simulink model "penduleBF"  (R2012b)
settings: Solver=ode45  StartTime=0.0  StopTime=15  MaxStep=0.01  RelTol=1e-3  AbsTol=1e-3
values from neighbouring files (symbols this model uses):
  Adc = Ad-(Bd*Kcd)-(Kod*Cd)    [Synthese_Obs_Contr_Pendule.m]
  Bdc = Kod    [Synthese_Obs_Contr_Pendule.m]
  Cdc = Kcd    [Synthese_Obs_Contr_Pendule.m]
  Ddc = [0,0]    [Synthese_Obs_Contr_Pendule.m]
  Tech = 0.01    [Synthese_Obs_Contr_Pendule.m]
settings Model: ExtModeTrigMode=oneshot  ExtModeArmWhenConnect=off  Creator=ArbenCela  LastModifiedBy=lalinden
settings DataIOCC: LimitDataPoints=off  SignalLoggingSaveFormat=ModelDataLogs  SaveOutput=off  SaveTime=off
settings OptimizationCC: BooleanDataType=off  ExpressionDepthLimit=128  InitFltsAndDblsToZero=on
settings DebuggingCC: SaveWithParameterizedLinksMsg=none  SignalResolutionControl=TryResolveAllWithWarning  SolverPrmCheckMsg=none  MultiTaskDSMMsg=warning  MultiTaskCondExecSysMsg=none  FcnCallInpInsideContextMsg=UseLocalSettings  StateNameClashWarn=none  StrictBusMsg=None
settings HardwareCC: TargetUnknown=on
settings RTWCC: IncludeERTFirstTime=on
settings CodeAppCC: CustomSymbolStrType=$N$R$M_T  InternalIdentifier=Shortened
settings GRTTargetCC: TargetFcnLib=ansi_tfl_tmw.mat  CodeReplacementLibrary=None  CombineOutputUpdateFcns=off  CPPClassGenCompliant=on  GRTInterface=on

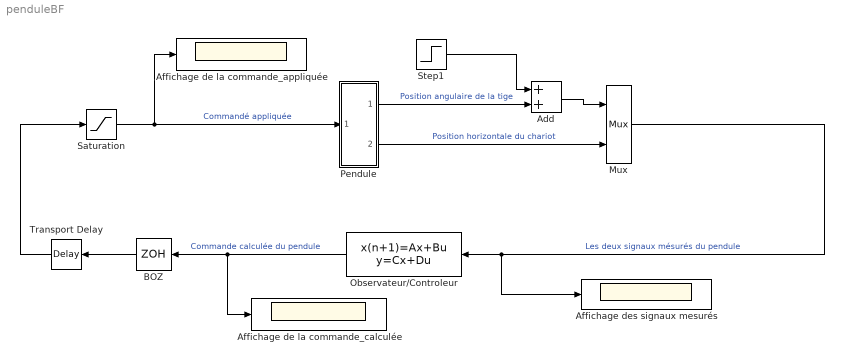
== system penduleBF ==
  Add : Sum
  Affichage de la commande_appliquée : Scope
      settings: YMin=2e+008  YMax=5.75e+008  SaveName=ScopeData2
  Affichage de la commande_calculée : Scope
      settings: YMin=2e+008  YMax=5.75e+008
  Affichage des signaux mesurés : Scope
      settings: YMin=-250000  YMax=1.75e+006
  BOZ : ZeroOrderHold  SampleTime=Tech
  Mux : Mux  Inputs=2
  Observateur/Controleur : DiscreteStateSpace  A=Adc  B=Bdc  C=-Cdc  D=Ddc  X0=[0;0;0;0]  SampleTime=Tech
  Pendule : Subsystem
  Saturation : Saturate  UpperLimit=10  LowerLimit=-10
  Step1 : Step  Time=2  After=0.02  SampleTime=0
  Transport Delay : TransportDelay  DelayTime=0.005
  wires:
  Pendule/2(out_2) -> Mux/2  "Position horizontale du chariot"
  Observateur/Controleur/1 -> Affichage de la commande_calculée/1, BOZ/1  "Commande calculée du pendule"
  Mux/1 -> Observateur/Controleur/1, Affichage des signaux mesurés/1  "Les deux signaux mésurés du pendule"
  Saturation/1 -> Pendule/1(in_1), Affichage de la commande_appliquée/1  "Commandé appliquée"
  Pendule/1(out_1) -> Add/2  "Position angulaire de la tige"
  Add/1 -> Mux/1
  BOZ/1 -> Transport Delay/1
  Transport Delay/1 -> Saturation/1
  Step1/1 -> Add/1

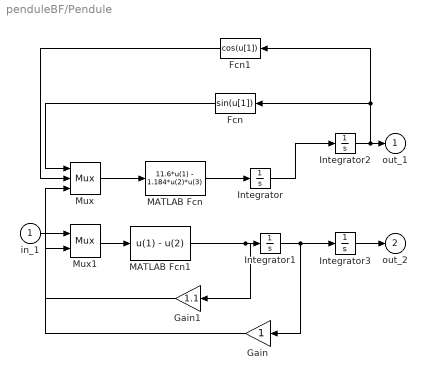
== system penduleBF/Pendule ==
  in_1 : Inport
  Fcn : Fcn
  Fcn1 : Fcn  Expr=cos(u[1])
  Gain : Gain  SaturateOnIntegerOverflow=on  OutDataTypeStr=Inherit: Same as input  ParamDataTypeStr=Inherit: Same as input
  Gain1 : Gain  Gain=1.1  SaturateOnIntegerOverflow=on  OutDataTypeStr=Inherit: Same as input  ParamDataTypeStr=Inherit: Same as input
  Integrator : Integrator
  Integrator1 : Integrator
  Integrator2 : Integrator  InitialCondition=0.1
  Integrator3 : Integrator
  MATLAB Fcn : MATLABFcn  MATLABFcn=11.6*u(1) - 1.184*u(2)*u(3)  OutputDimensions=1
  MATLAB Fcn1 : MATLABFcn  MATLABFcn=u(1) - u(2)  OutputDimensions=1
  Mux : Mux  Inputs=3
  Mux1 : Mux  Inputs=2
  out_1 : Outport
  out_2 : Outport  Port=2
  wires:
  Integrator/1 -> Integrator2/1
  Integrator2/1 -> Fcn/1, Fcn1/1, out_1/1
  Fcn/1 -> Mux/1
  Fcn1/1 -> Mux/2
  Mux1/1 -> MATLAB Fcn1/1
  Mux/1 -> MATLAB Fcn/1
  MATLAB Fcn/1 -> Integrator/1
  MATLAB Fcn1/1 -> Integrator1/1, Gain1/1
  Gain1/1 -> Mux/3
  Gain/1 -> Mux1/2
  Integrator1/1 -> Integrator3/1, Gain/1
  in_1/1 -> Mux1/1
  Integrator3/1 -> out_2/1
